simulink subsystem "EPS_Physical_Model"  (R2024a)
settings: Solver=VariableStepAuto  StartTime=0.0  StopTime=10.0  RelTol=1e-3
undefined symbols (not defined in the file): dcVoltage, Power, satellite, sensor
libraries: nesl_utility x25, fl_lib x24, ee_lib x6, autolibdatasheetbattery x1
(part 1 of 2)
settings Model: Creator=dani  LastModifiedBy=dani

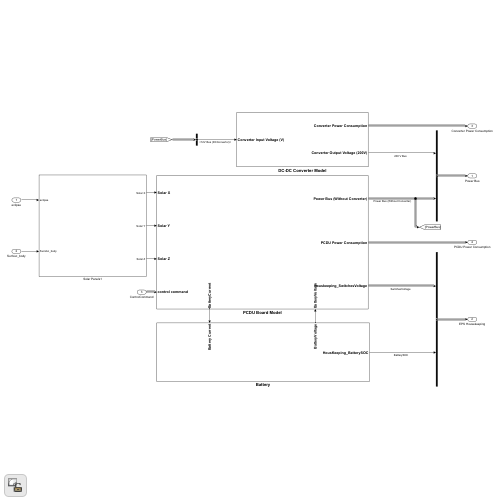
[thumbnail: Simulink's stored preview of the top-level diagram]
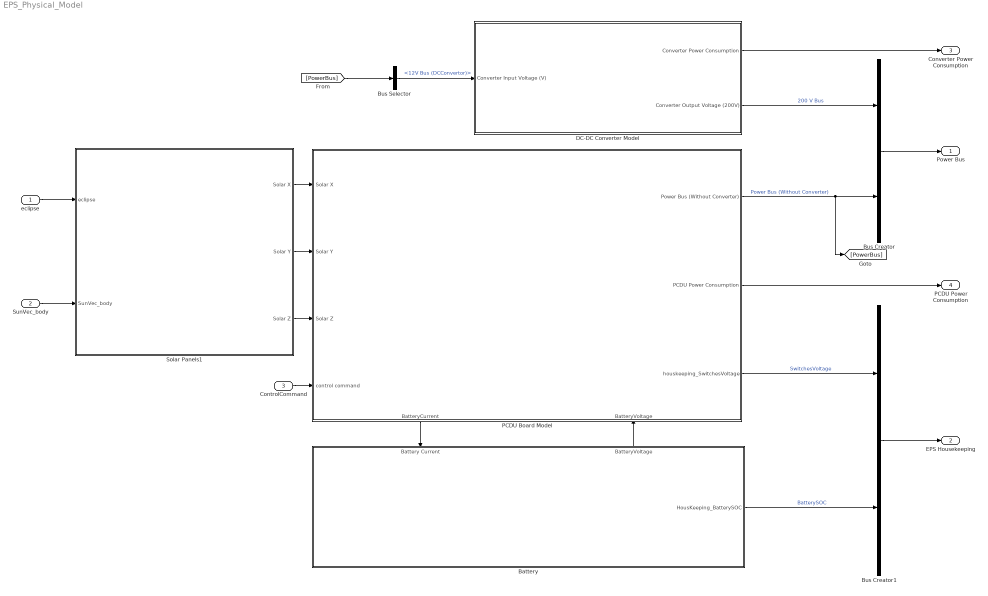
== system EPS_Physical_Model ==
  eclipse : Inport
  SunVec_body : Inport  Port=2
  ControlCommand : Inport  Port=3
  Battery : Subsystem
      settings: PortSchema="{\"entries\":[{\"content\":{\"sides\":[{\"content\":{},\"type\":\"ConnectorPlacement.EquallySpacedRectSide\",\"uuid\":\"aba023eb-c61a-4f67-b0b4-9861c526ec15\"},{\"content\":{\"connectorIds\":[\"Out1\"],\"side\":\"RIGHT\"},\"type\":\"ConnectorPlacement.EquallySpacedRectSide\",\"uuid\":\"3f6535be-9be1-4768-b763-1183b5aa3573\"},{\"content\":{\"connectorIds\":[\"In1\",\"Out2\"],\"side\":\"TOP\"},\"type\":\"ConnectorPlacement.EquallySpacedRectSide\",\"uuid\":\"4513aba4-b806-45fb-9bac-31582bd0c290\"}]},\"type\":\"ConnectorPlacement.EquallySpacedConnector\",\"uuid\":\"e35f9ef2-784c-4297-8a3a-3364ea15e971\"}],\"packageUris\":[\"http://schema.mathworks.com/mf0/Connector/R2020b\"],\"version\":\"1.0\"}"
  Bus Creator : BusCreator  Inputs=2
  Bus Creator1 : BusCreator  Inputs=2
  Bus Selector : BusSelector  OutputSignals=12V Bus (DCConvertor)
  DC-DC Converter Model : Subsystem
  PCDU Board Model : Subsystem
      settings: PortSchema="{\"entries\":[{\"content\":{\"sides\":[{\"content\":{\"connectorIds\":[\"In1\",\"In2\",\"In3\",\"In4\"]},\"type\":\"ConnectorPlacement.EquallySpacedRectSide\",\"uuid\":\"36672ca7-eb13-4725-b00c-09a487ba7d91\"},{\"content\":{\"connectorIds\":[\"Out1\",\"Out2\",\"Out3\"],\"side\":\"RIGHT\"},\"type\":\"ConnectorPlacement.EquallySpacedRectSide\",\"uuid\":\"6eafcdb3-9ad1-4020-b7cb-384bf41fe7fc\"},{\"content\":{\"side\":\"TOP\"},\"type\":\"ConnectorPlacement.EquallySpacedRectSide\",\"uuid\":\"e91cfa27-9882-4a24-903a-d0e72077027b\"},{\"content\":{\"connectorIds\":[\"Out4\",\"In5\"],\"side\":\"BOTTOM\"},\"type\":\"ConnectorPlacement.EquallySpacedRectSide\",\"uuid\":\"cff8a778-7a2c-4410-b33c-165bd9362bc6\"}]},\"type\":\"ConnectorPlacement.EquallySpacedConnector\",\"uuid\":\"92ed5259-46ff-4d91-b4a9-1e7fd77d238d\"}],\"packageUris\":[\"http://schema.mathworks.com/mf0/Connector/R2020b\"],\"version\":\"1.0\"}"
  Solar Panels1 : Subsystem
  Power Bus : Outport
  EPS Housekeeping : Outport  Port=2
  Converter Power Consumption : Outport  Port=3
  PCDU Power Consumption : Outport  Port=4
  wires:
  eclipse/1 -> Solar Panels1/1(eclipse)
  Solar Panels1/1(Solar X) -> PCDU Board Model/1(Solar X)
  Solar Panels1/2(Solar Y) -> PCDU Board Model/2(Solar Y)
  Solar Panels1/3(Solar Z) -> PCDU Board Model/3(Solar Z)
  Bus Creator/1 -> Power Bus/1
  Bus Creator1/1 -> EPS Housekeeping/1
  ControlCommand/1 -> PCDU Board Model/4(control command)
  SunVec_body/1 -> Solar Panels1/2(SunVec_body)
  PCDU Board Model/1(Power Bus (Without Converter)) -> Bus Creator/2, [PowerBus]  "Power Bus (Without Converter)"
  PCDU Board Model/4(BatteryCurrent) -> Battery/1(Battery Current)
  Battery/2(BatteryVoltage) -> PCDU Board Model/5(BatteryVoltage)
  Bus Selector/1 -> DC-DC Converter Model/1(Converter Input Voltage (V))  "<12V Bus (DCConvertor)>"
  PCDU Board Model/3(houskeeping_SwitchesVoltage) -> Bus Creator1/1  "SwitchesVoltage"
  Battery/1(HousKeeping_BatterySOC) -> Bus Creator1/2  "BatterySOC"
  [PowerBus] -> Bus Selector/1
  DC-DC Converter Model/1(Converter Power Consumption) -> Converter Power Consumption/1
  PCDU Board Model/2(PCDU Power Consumption) -> PCDU Power Consumption/1
  DC-DC Converter Model/2(Converter Output Voltage (200V)) -> Bus Creator/1  "200 V Bus"

== system EPS_Physical_Model/Battery ==
  Battery Current : Inport
  Bus Selector : BusSelector  OutputSignals=BattSoc
  Constant : Constant  Value=275
  Lithium Polymer Battery Pack : autolibdatasheetbattery/Datasheet Battery  CapacityCtrl=Parameter  OutputVlt=Unfiltered  BattChargeMax=100  Em=[2.8 3.228 3.284 3.361 3.408 3.427 3.472 3.477 3.493 3.504 3.516 3.528 3.537 3.545 3.555 3.561 3.566 3.576 3.587 3.589 3.594 3.6 3.608 3.61 3.616 3.619 3.626 3.632 3.637 3.64 3.645 3.646 3.652 3.655 3.658 3.661 3.664 3.668 3.673 3.678 3.68 3.681 3.686 3.692 3.699 3.702 3.705 3.71 3.717 3.723 3.728 3.733 3.735 3.742 3.749 3.755 3.761 3.768 3.773 3.78 3.791 3.798 3.798 3.814 3.818 3.825 3.841 3.846 3.855 3.863 3.877 3.885 3.894 3.907 3.919 3.926 3.935 3.944 3.954 3.964 3.974 3.988 3.998 4.014 4.029 4.034 4.047 4.065 4.074 4.086 4.097 4.131 4.126 4.138 4.15 4.18 4.174 4.187 4.207 4.231 4.221]  CapLUTBp=[0 0.01 0.02 0.03 0.04 0.05 0.06 0.07 0.08 0.09 0.1 0.11 0.12 0.13 0.14 0.15 0.16 0.17 0.18 0.19 0.2 0.21 0.22 0.23 0.24 0.25 0.26 0.27 0.28 0.29 0.3 0.31 0.32 0.33 0.34 0.35 0.36 0.37 0.38 0.39 0.4 0.41 0.42 0.43 0.44 0.45 0.46 0.47 0.48 0.49 0.5 0.51 0.52 0.53 0.54 0.55 0.56 0.57 0.58 0.59 0.6 0.61 0.62 0.63 0.64 0.65 0.66 0.67 0.68 0.69 0.7 0.71 0.72 0.73 0.74 0.75 0.76 0.77 0.78 0.79 0.8 0.81 0.82 0.83 0.84 0.85 0.86 0.87 0.88 0.89 0.9 0.91 0.92 0.93 0.94 0.95 0.96 0.97 0.98 0.99 1]  RInt=[0.008846 0.009319 0.009027 0.00847 0.01032 0.01314;0.006389 0.006554 0.005553 0.005525 0.006043 0.007805;0.004364 0.004101 0.00406 0.003452 0.003846 0.004517;0.002031 0.002563 0.002532 0.00246 0.002716 0.003047;0.001443 0.001825 0.001795 0.001778 0.001924 0.002234;0.0005603 0.0007192 0.0006887 0.0007557 0.0007355 0.001014;0.001028 0.001338 0.001 0.001536 0.001546 0.002789]  BattTempBp=[243.1 253.1 263.1 273.1 283.1 298.1 313.1]  CapSOCBp=[0 0.2 0.4 0.6 0.8 1]  Ns=1  Np=1  BattCapInit=100  Tc=1/1000  Vinit=4.221  RefBlkName='autolibdatasheetbattery/Datasheet Battery'
  HousKeeping_BatterySOC : Outport
  BatteryVoltage : Outport  Port=2
  wires:
  Lithium Polymer Battery Pack/2 -> BatteryVoltage/1
  Constant/1 -> Lithium Polymer Battery Pack/2
  Bus Selector/1 -> HousKeeping_BatterySOC/1  "<BattSoc>"
  Battery Current/1 -> Lithium Polymer Battery Pack/1
  Lithium Polymer Battery Pack/1 -> Bus Selector/1

== system EPS_Physical_Model/DC-DC Converter Model ==
  Converter Input Voltage (V) : Inport
  Constant : Constant  Value=satellite.Converter.OutputVoltage
  Divide : Product  Inputs=*/
  Power Consumption Calculator : Subsystem
  Product : Product
  Terminator : Terminator
  Converter Power Consumption : Outport
  Converter Output Voltage (200V) : Outport  Port=2
  wires:
  Constant/1 -> Divide/1, Converter Output Voltage (200V)/1
  Product/1 -> Terminator/1
  Power Consumption Calculator/1(Power Consumption) -> Converter Power Consumption/1
  Divide/1 -> Product/1
  Converter Input Voltage (V)/1 -> Power Consumption Calculator/1(Bus Voltage (V)), Divide/2, Product/2

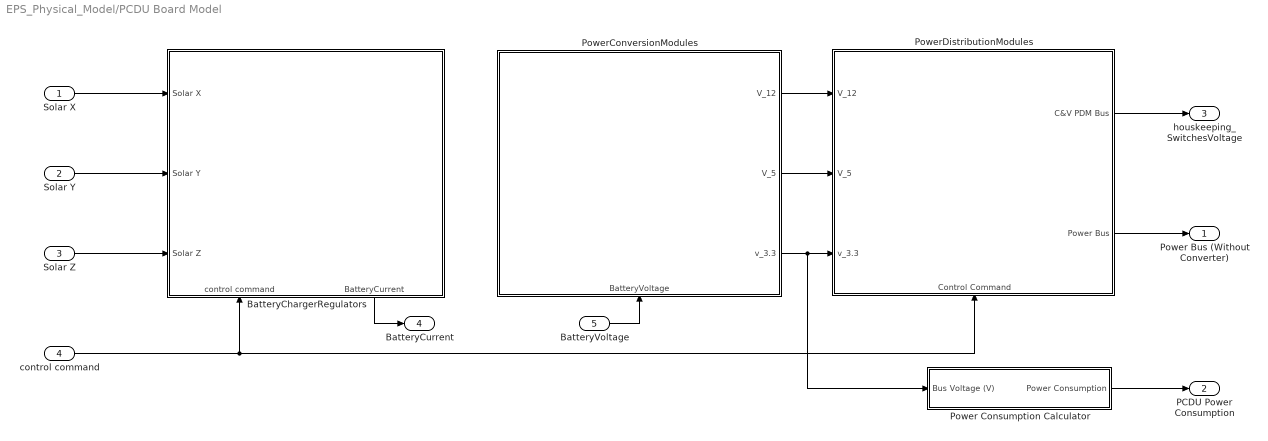
== system EPS_Physical_Model/PCDU Board Model ==
  Solar X : Inport
  Solar Y : Inport  Port=2
  Solar Z : Inport  Port=3
  control command : Inport  Port=4
  BatteryVoltage : Inport  Port=5
  BatteryChargerRegulators : Subsystem
      settings: PortSchema="{\"entries\":[{\"content\":{\"sides\":[{\"content\":{\"connectorIds\":[\"In1\",\"In2\",\"In3\"]},\"type\":\"ConnectorPlacement.EquallySpacedRectSide\",\"uuid\":\"a54c6477-f532-403d-8d22-fe8c7187031b\"},{\"content\":{\"side\":\"RIGHT\"},\"type\":\"ConnectorPlacement.EquallySpacedRectSide\",\"uuid\":\"77a78f68-d33d-41d0-b8f1-9e3ab7c3612b\"},{\"content\":{\"side\":\"TOP\"},\"type\":\"ConnectorPlacement.EquallySpacedRectSide\",\"uuid\":\"40e6fe94-fdf3-42ac-b4f7-43c530d7ca8e\"},{\"content\":{\"connectorIds\":[\"In4\",\"Out1\"],\"side\":\"BOTTOM\"},\"type\":\"ConnectorPlacement.EquallySpacedRectSide\",\"uuid\":\"5f994662-38e6-4570-aab0-67fb9122f990\"}]},\"type\":\"ConnectorPlacement.EquallySpacedConnector\",\"uuid\":\"6ae65874-5838-4158-9d12-5770a4409470\"}],\"packageUris\":[\"http://schema.mathworks.com/mf0/Connector/R2020b\"],\"version\":\"1.0\"}"
  Power Consumption Calculator : Subsystem
  PowerConversionModules : Subsystem
      settings: PortSchema="{\"entries\":[{\"content\":{\"sides\":[{\"content\":{},\"type\":\"ConnectorPlacement.EquallySpacedRectSide\",\"uuid\":\"7faa42b3-e758-4a59-bd59-cf39d4aa9549\"},{\"content\":{\"connectorIds\":[\"Out1\",\"Out2\",\"Out3\"],\"side\":\"RIGHT\"},\"type\":\"ConnectorPlacement.EquallySpacedRectSide\",\"uuid\":\"fd6f184d-0914-459d-a4a5-5106acefe1a2\"},{\"content\":{\"side\":\"TOP\"},\"type\":\"ConnectorPlacement.EquallySpacedRectSide\",\"uuid\":\"8eb7f5a0-03ff-41d6-8f99-6dc2709a1a61\"},{\"content\":{\"connectorIds\":[\"In1\"],\"side\":\"BOTTOM\"},\"type\":\"ConnectorPlacement.EquallySpacedRectSide\",\"uuid\":\"52483d8d-c391-40d7-8f9f-4b93cbeba715\"}]},\"type\":\"ConnectorPlacement.EquallySpacedConnector\",\"uuid\":\"8e205f56-f28b-497f-b412-2c567253f0db\"}],\"packageUris\":[\"http://schema.mathworks.com/mf0/Connector/R2020b\"],\"version\":\"1.0\"}"
  PowerDistributionModules : Subsystem
      settings: PortSchema="{\"entries\":[{\"content\":{\"sides\":[{\"content\":{\"connectorIds\":[\"In1\",\"In2\",\"In3\"]},\"type\":\"ConnectorPlacement.EquallySpacedRectSide\",\"uuid\":\"cc944067-0ae4-44c1-82d9-a1ec81fe8cae\"},{\"content\":{\"connectorIds\":[\"Out1\",\"Out2\"],\"side\":\"RIGHT\"},\"type\":\"ConnectorPlacement.EquallySpacedRectSide\",\"uuid\":\"14a8b3bc-9f23-4806-a571-fc273ce75e66\"},{\"content\":{\"side\":\"TOP\"},\"type\":\"ConnectorPlacement.EquallySpacedRectSide\",\"uuid\":\"d74dfaa3-3ba0-49fd-a7b0-c7f12b34c19f\"},{\"content\":{\"connectorIds\":[\"In4\"],\"side\":\"BOTTOM\"},\"type\":\"ConnectorPlacement.EquallySpacedRectSide\",\"uuid\":\"4657f579-020f-4b4b-b590-abcb58cae511\"}]},\"type\":\"ConnectorPlacement.EquallySpacedConnector\",\"uuid\":\"36922770-3f3d-4d84-84df-ae2b6fb05eab\"}],\"packageUris\":[\"http://schema.mathworks.com/mf0/Connector/R2020b\"],\"version\":\"1.0\"}"
  Power Bus (Without Converter) : Outport
  PCDU Power Consumption : Outport  Port=2
  houskeeping_SwitchesVoltage : Outport  Port=3
  BatteryCurrent : Outport  Port=4
  wires:
  control command/1 -> BatteryChargerRegulators/4(control command), PowerDistributionModules/4(Control Command)
  PowerConversionModules/2(V_5) -> PowerDistributionModules/2(V_5)
  PowerConversionModules/1(V_12) -> PowerDistributionModules/1(V_12)
  BatteryVoltage/1 -> PowerConversionModules/1(BatteryVoltage)
  PowerConversionModules/3(v_3.3) -> PowerDistributionModules/3(v_3.3), Power Consumption Calculator/1(Bus Voltage (V))
  BatteryChargerRegulators/1(BatteryCurrent) -> BatteryCurrent/1
  Power Consumption Calculator/1(Power Consumption) -> PCDU Power Consumption/1
  PowerDistributionModules/1(C&V PDM Bus) -> houskeeping_SwitchesVoltage/1
  Solar Y/1 -> BatteryChargerRegulators/2(Solar Y)
  PowerDistributionModules/2(Power Bus) -> Power Bus (Without Converter)/1
  Solar Z/1 -> BatteryChargerRegulators/3(Solar Z)
  Solar X/1 -> BatteryChargerRegulators/1(Solar X)

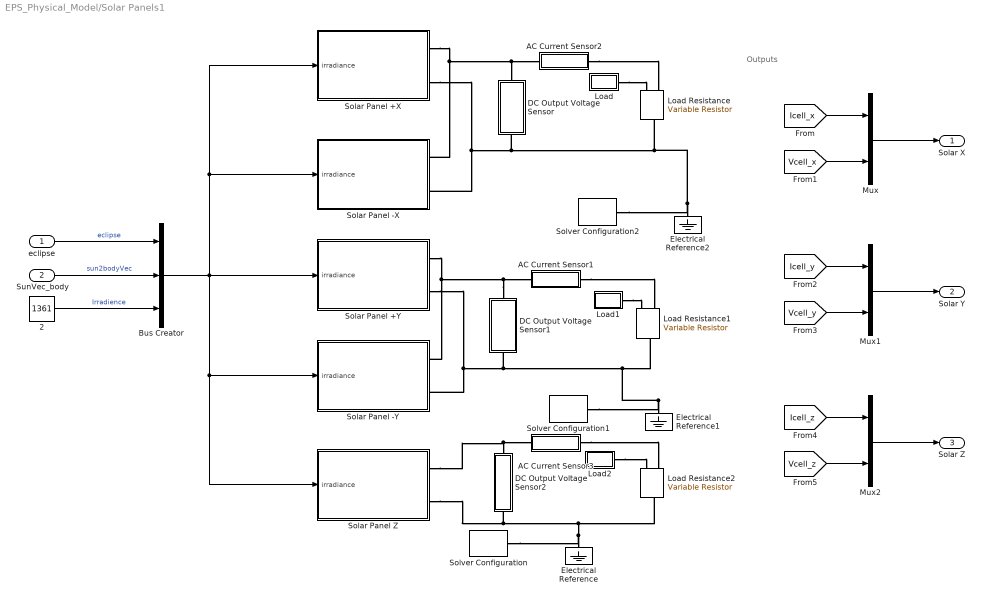
== system EPS_Physical_Model/Solar Panels1 ==
  note: Outputs
  eclipse : Inport
  SunVec_body : Inport  Port=2
  " 2" : Constant  Value=1361
  AC Current Sensor1 : Subsystem
      mask Display: disp('i');
  AC Current Sensor2 : Subsystem
      mask Display: disp('i');
  AC Current Sensor3 : Subsystem
      mask Display: disp('i');
  Bus Creator : BusCreator  Inputs=3
  DC Output Voltage Sensor : Subsystem
      mask Display: disp('v')
  DC Output Voltage Sensor1 : Subsystem
      mask Display: disp('v')
  DC Output Voltage Sensor2 : Subsystem
      mask Display: disp('v')
  Electrical Reference : fl_lib/Electrical/Electrical Elements/Electrical Reference
  Electrical Reference1 : fl_lib/Electrical/Electrical Elements/Electrical Reference
  Electrical Reference2 : fl_lib/Electrical/Electrical Elements/Electrical Reference
  Load : Subsystem
  Load Resistance : fl_lib/Electrical/Electrical Elements/Variable Resistor  Rmin=0 Ohm  thermalEnable=false  thermal_mass=1 J/K  i_specify=off  i_priority=None  i=5 A  i_nominal_specify=off  i_nominal_value=1  i_nominal_unit=A  v_specify=off  v_priority=None  v=0 V  v_nominal_specify=off  v_nominal_value=1  v_nominal_unit=V  T_specify=off  T_priority=None  T=300 K  T_nominal_specify=off  T_nominal_value=1  T_nominal_unit=K
  Load Resistance1 : fl_lib/Electrical/Electrical Elements/Variable Resistor  Rmin=0 Ohm  thermalEnable=false  thermal_mass=1 J/K  i_specify=off  i_priority=None  i=5 A  i_nominal_specify=off  i_nominal_value=1  i_nominal_unit=A  v_specify=off  v_priority=None  v=0 V  v_nominal_specify=off  v_nominal_value=1  v_nominal_unit=V  T_specify=off  T_priority=None  T=300 K  T_nominal_specify=off  T_nominal_value=1  T_nominal_unit=K
  Load Resistance2 : fl_lib/Electrical/Electrical Elements/Variable Resistor  Rmin=0 Ohm  thermalEnable=false  thermal_mass=1 J/K  i_specify=off  i_priority=None  i=5 A  i_nominal_specify=off  i_nominal_value=1  i_nominal_unit=A  v_specify=off  v_priority=None  v=0 V  v_nominal_specify=off  v_nominal_value=1  v_nominal_unit=V  T_specify=off  T_priority=None  T=300 K  T_nominal_specify=off  T_nominal_value=1  T_nominal_unit=K
  Load1 : Subsystem
  Load2 : Subsystem
  Mux : Mux  Inputs=2
  Mux1 : Mux  Inputs=2
  Mux2 : Mux  Inputs=2
  Solar Panel +X : Subsystem
  Solar Panel +Y : Subsystem
  Solar Panel -X : Subsystem
  Solar Panel -Y : Subsystem
  Solar Panel Z : Subsystem
  Solver Configuration : nesl_utility/Solver Configuration  PhysicalDomain=network_engine_domain  SubClassName=solver  LeftPortType=input  RightPortType=generic  Tones=[]  Harmonics=[]  SimulateNoise=off  Profile=off  UseLocalSampling=off  EnableSwitchedLinearOptims=on  FrequencyDomain=off  UseCCode=off  RelTol=0.001  AbsTol=0.001  MinStep=1e-09  ToWorkspace=off  RevertToSquareIcSolve=off  NumHomotopyIterations=100  PhasorMode=off  PhasorModeNumHarmonics=1  ConsistencySolver=NEWTON_XTOL_AFTER_FTOL  IndexReductionMethod=DerivativeReplacement  DoDC=off  ResidualTolerance=1e-09  ConsistencyTolSource=GLOBAL  ConsistencyAbsTol=0.001  ConsistencyRelTol=0.001  ConsistencyTolFactor=0.001  UseLocalSolver=off  LocalSolverChoice=NE_BACKWARD_EULER_ADVANCER  ResolveIndetEquations=on  FunctionEvalNumThread=1  LocalSolverSampleTime=0.001  DoFixedCost=off  MaxNonlinIter=3  MaxModeIter=2  ComputeImpulses=off  ImpulseIterations=2  LinearAlgebra=auto  LinearAlgebraNumThread=0  EquationFormulation=NE_TIME_EF  DelaysMemoryBudget=1024  AutomaticFiltering=on  FilteringTimeConstant=0.001  PartitionStorageMethod=AS_NEEDED  PartitionMemoryBudget=1024  PartitionMethod=ROBUST  MultibodyUseLocalSolver=off  MultibodyLocalSolverChoice=ODE1  MultibodyLocalSolverSampleTime=0.001
  Solver Configuration1 : nesl_utility/Solver Configuration  PhysicalDomain=network_engine_domain  SubClassName=solver  LeftPortType=input  RightPortType=generic  Tones=[]  Harmonics=[]  SimulateNoise=off  Profile=off  UseLocalSampling=off  EnableSwitchedLinearOptims=on  FrequencyDomain=off  UseCCode=off  RelTol=0.001  AbsTol=0.001  MinStep=1e-09  ToWorkspace=off  RevertToSquareIcSolve=off  NumHomotopyIterations=100  PhasorMode=off  PhasorModeNumHarmonics=1  ConsistencySolver=NEWTON_XTOL_AFTER_FTOL  IndexReductionMethod=DerivativeReplacement  DoDC=off  ResidualTolerance=1e-09  ConsistencyTolSource=GLOBAL  ConsistencyAbsTol=0.001  ConsistencyRelTol=0.001  ConsistencyTolFactor=0.001  UseLocalSolver=off  LocalSolverChoice=NE_BACKWARD_EULER_ADVANCER  ResolveIndetEquations=on  FunctionEvalNumThread=1  LocalSolverSampleTime=0.001  DoFixedCost=off  MaxNonlinIter=3  MaxModeIter=2  ComputeImpulses=off  ImpulseIterations=2  LinearAlgebra=auto  LinearAlgebraNumThread=0  EquationFormulation=NE_TIME_EF  DelaysMemoryBudget=1024  AutomaticFiltering=on  FilteringTimeConstant=0.001  PartitionStorageMethod=AS_NEEDED  PartitionMemoryBudget=1024  PartitionMethod=ROBUST  MultibodyUseLocalSolver=off  MultibodyLocalSolverChoice=ODE1  MultibodyLocalSolverSampleTime=0.001
  Solver Configuration2 : nesl_utility/Solver Configuration  PhysicalDomain=network_engine_domain  SubClassName=solver  LeftPortType=input  RightPortType=generic  Tones=[]  Harmonics=[]  SimulateNoise=off  Profile=off  UseLocalSampling=off  EnableSwitchedLinearOptims=on  FrequencyDomain=off  UseCCode=off  RelTol=0.001  AbsTol=0.001  MinStep=1e-09  ToWorkspace=off  RevertToSquareIcSolve=off  NumHomotopyIterations=100  PhasorMode=off  PhasorModeNumHarmonics=1  ConsistencySolver=NEWTON_XTOL_AFTER_FTOL  IndexReductionMethod=DerivativeReplacement  DoDC=off  ResidualTolerance=1e-09  ConsistencyTolSource=GLOBAL  ConsistencyAbsTol=0.001  ConsistencyRelTol=0.001  ConsistencyTolFactor=0.001  UseLocalSolver=off  LocalSolverChoice=NE_BACKWARD_EULER_ADVANCER  ResolveIndetEquations=on  FunctionEvalNumThread=1  LocalSolverSampleTime=0.001  DoFixedCost=off  MaxNonlinIter=3  MaxModeIter=2  ComputeImpulses=off  ImpulseIterations=2  LinearAlgebra=auto  LinearAlgebraNumThread=0  EquationFormulation=NE_TIME_EF  DelaysMemoryBudget=1024  AutomaticFiltering=on  FilteringTimeConstant=0.001  PartitionStorageMethod=AS_NEEDED  PartitionMemoryBudget=1024  PartitionMethod=ROBUST  MultibodyUseLocalSolver=off  MultibodyLocalSolverChoice=ODE1  MultibodyLocalSolverSampleTime=0.001
  Solar X : Outport
  Solar Y : Outport  Port=2
  Solar Z : Outport  Port=3
  wires:
  SunVec_body/1 -> Bus Creator/2  "sun2bodyVec"
  eclipse/1 -> Bus Creator/1  "eclipse"
  " 2"/1 -> Bus Creator/3  "Irradience"
  Mux1/1 -> Solar Y/1
  Mux2/1 -> Solar Z/1
  Mux/1 -> Solar X/1
  [Vcell_z] -> Mux2/2
  [Icell_z] -> Mux2/1
  [Icell_x] -> Mux/1
  [Vcell_x] -> Mux/2
  [Icell_y] -> Mux1/1
  [Vcell_y] -> Mux1/2
  Bus Creator/1 -> Solar Panel +Y/1(irradiance), Solar Panel Z/1(irradiance), Solar Panel -Y/1(irradiance), Solar Panel +X/1(irradiance), Solar Panel -X/1(irradiance)
  connections:
  AC Current Sensor2/LConn1 -- Load Resistance/LConn2
  Load1/RConn1 -- Load Resistance1/LConn1
  Load2/RConn1 -- Load Resistance2/LConn1
  AC Current Sensor1/LConn1 -- Load Resistance1/LConn2
  Load/RConn1 -- Load Resistance/LConn1
  AC Current Sensor3/LConn1 -- Load Resistance2/LConn2
  DC Output Voltage Sensor2/RConn1 -- Solar Panel Z/RConn1 -- AC Current Sensor3/RConn1
  Solver Configuration1/RConn1 -- DC Output Voltage Sensor1/LConn1 -- Solar Panel -Y/RConn2 -- Solar Panel +Y/RConn2 -- Load Resistance1/RConn1 -- Electrical Reference1/LConn1
  Load Resistance2/RConn1 -- Electrical Reference/LConn1 -- Solver Configuration/RConn1 -- Solar Panel Z/RConn2 -- DC Output Voltage Sensor2/LConn1
  Solar Panel -X/RConn1 -- Solar Panel +X/RConn1 -- AC Current Sensor2/RConn1 -- DC Output Voltage Sensor/RConn1
  Solver Configuration2/RConn1 -- Load Resistance/RConn1 -- Solar Panel -X/RConn2 -- Solar Panel +X/RConn2 -- DC Output Voltage Sensor/LConn1 -- Electrical Reference2/LConn1
  DC Output Voltage Sensor1/RConn1 -- AC Current Sensor1/RConn1 -- Solar Panel -Y/RConn1 -- Solar Panel +Y/RConn1

== system EPS_Physical_Model/DC-DC Converter Model/Power Consumption Calculator ==
  note: $I_=\frac{V_{Bus}}{R} \\ P_{Consumption} =I V_{Bus}$
  Bus Voltage (V) : Inport
  1/R : Gain  Gain=1/Power.Converter.Resistance
  Bus Creator : BusCreator  Inputs=2
  Product : Product
  Power Consumption : Outport
  wires:
  Product/1 -> Bus Creator/2  "Power Consumption (W)"
  Bus Creator/1 -> Power Consumption/1
  1/R/1 -> Bus Creator/1, Product/1  "Current (A)"
  Bus Voltage (V)/1 -> 1/R/1, Product/2

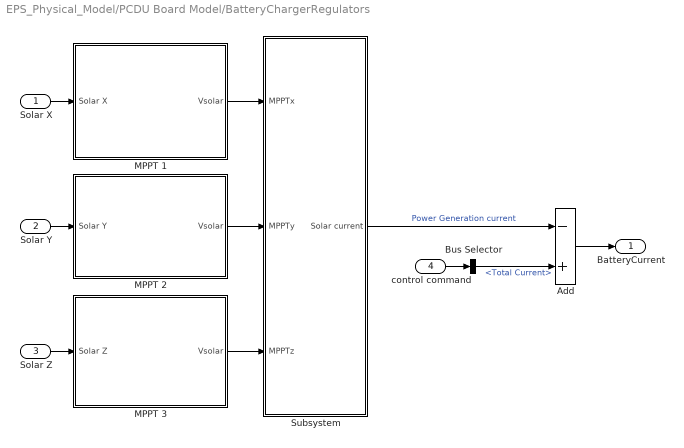
== system EPS_Physical_Model/PCDU Board Model/BatteryChargerRegulators ==
  Solar X : Inport
  Solar Y : Inport  Port=2
  Solar Z : Inport  Port=3
  control command : Inport  Port=4
  Add : Sum  Inputs=-+
  Bus Selector : BusSelector  OutputSignals=Total Current
  MPPT 1 : Subsystem
  MPPT 2 : Subsystem
  MPPT 3 : Subsystem
  Subsystem : Subsystem
  BatteryCurrent : Outport
  wires:
  control command/1 -> Bus Selector/1
  Bus Selector/1 -> Add/2  "<Total Current>"
  Solar Z/1 -> MPPT 3/1(Solar Z)
  Solar X/1 -> MPPT 1/1(Solar X)
  MPPT 3/1(Vsolar) -> Subsystem/3(MPPTz)
  Subsystem/1(Solar current) -> Add/1  "Power Generation current"
  Solar Y/1 -> MPPT 2/1(Solar Y)
  MPPT 1/1(Vsolar) -> Subsystem/1(MPPTx)
  Add/1 -> BatteryCurrent/1
  MPPT 2/1(Vsolar) -> Subsystem/2(MPPTy)

== system EPS_Physical_Model/PCDU Board Model/Power Consumption Calculator ==
  note: $I_=\frac{V_{Bus}}{R} \\ P_{Consumption} =I V_{Bus}$
  Bus Voltage (V) : Inport
  1/R : Gain  Gain=1/Power.PCDU.Resistance
  Bus Creator : BusCreator  Inputs=2
  Product : Product
  Power Consumption : Outport
  wires:
  Product/1 -> Bus Creator/2  "Power Consumption (W)"
  Bus Creator/1 -> Power Consumption/1
  1/R/1 -> Bus Creator/1, Product/1  "Current (A)"
  Bus Voltage (V)/1 -> 1/R/1, Product/2

== system EPS_Physical_Model/PCDU Board Model/PowerConversionModules ==
  BatteryVoltage : Inport
  Boost_12V : Subsystem
  Boost_3.3V : Subsystem
  Boost_5V : Subsystem
  V_12 : Outport
  V_5 : Outport  Port=2
  v_3.3 : Outport  Port=3
  wires:
  Boost_3.3V/1(12V) -> v_3.3/1
  Boost_5V/1(12V) -> V_5/1
  Boost_12V/1(12V) -> V_12/1
  BatteryVoltage/1 -> Boost_5V/1(BatteryVoltage), Boost_3.3V/1(BatteryVoltage), Boost_12V/1(BatteryVoltage)

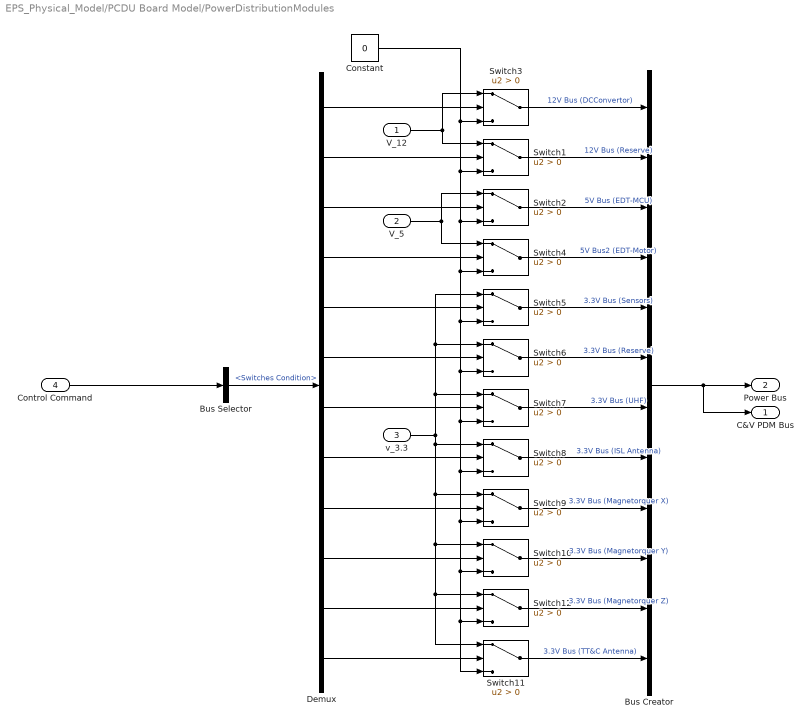
== system EPS_Physical_Model/PCDU Board Model/PowerDistributionModules ==
  V_12 : Inport
  V_5 : Inport  Port=2
  v_3.3 : Inport  Port=3
  Control Command : Inport  Port=4
  Bus Creator : BusCreator  Inputs=12
  Bus Selector : BusSelector  OutputSignals=Switches Condition
  Constant : Constant  Value=0
  Demux : Demux  Outputs=12
  Switch{1..12} (12 alike) : Switch  Criteria=u2 > Threshold  SaturateOnIntegerOverflow=off  InputSameDT=off
  C&V PDM Bus : Outport
  Power Bus : Outport  Port=2
  wires:
  Bus Selector/1 -> Demux/1  "<Switches Condition>"
  Demux/12 -> Switch11/2
  Demux/11 -> Switch12/2
  Demux/10 -> Switch10/2
  Demux/9 -> Switch9/2
  Demux/8 -> Switch8/2
  Demux/7 -> Switch7/2
  Demux/6 -> Switch6/2
  Demux/5 -> Switch5/2
  Demux/4 -> Switch4/2
  Demux/3 -> Switch2/2
  Demux/2 -> Switch1/2
  Demux/1 -> Switch3/2
  Bus Creator/1 -> C&V PDM Bus/1, Power Bus/1
  Switch11/1 -> Bus Creator/12  "3.3V Bus (TT&C Antenna)"
  Switch12/1 -> Bus Creator/11  "3.3V Bus (Magnetorquer Z)"
  Switch10/1 -> Bus Creator/10  "3.3V Bus (Magnetorquer Y)"
  Switch9/1 -> Bus Creator/9  "3.3V Bus (Magnetorquer X)"
  Switch8/1 -> Bus Creator/8  "3.3V Bus (ISL Antenna)"
  Switch7/1 -> Bus Creator/7  "3.3V Bus (UHF)"
  Switch6/1 -> Bus Creator/6  "3.3V Bus (Reserve)"
  Switch5/1 -> Bus Creator/5  "3.3V Bus (Sensors)"
  Switch4/1 -> Bus Creator/4  "5V Bus2 (EDT-Motor)"
  Switch2/1 -> Bus Creator/3  "5V Bus (EDT-MCU)"
  Switch1/1 -> Bus Creator/2  "12V Bus (Reserve)"
  Switch3/1 -> Bus Creator/1  "12V Bus (DCConvertor)"
  v_3.3/1 -> Switch8/1, Switch9/1, Switch10/1, Switch12/1, Switch11/1, Switch5/1, Switch6/1, Switch7/1
  V_5/1 -> Switch2/1, Switch4/1
  V_12/1 -> Switch3/1, Switch1/1
  Control Command/1 -> Bus Selector/1
  Constant/1 -> Switch3/3, Switch1/3, Switch2/3, Switch4/3, Switch5/3, Switch6/3, Switch7/3, Switch8/3, Switch9/3, Switch10/3, Switch12/3, Switch11/3

== system EPS_Physical_Model/Solar Panels1/AC Current Sensor1 ==
  Current Sensor : fl_lib/Electrical/Electrical Sensors/Current Sensor
  PS-Simulink Converter : nesl_utility/PS-Simulink Converter  PhysicalDomain=network_engine_domain  SubClassName=ps_output  LeftPortType=input  RightPortType=output  PseudoPeriodic=off  Frequencies=[]  VectorFormat=1-D array  Unit=1  AffineConversion=off
  Sensor dynamics : TransferFcn  Numerator=1  Denominator=[1 1]
  - : PMIOPort  Side=Left
  + : PMIOPort  Port=2  Side=Right
  tag scope: Icell_y=global
  wires:
  PS-Simulink Converter/1 -> Sensor dynamics/1
  Sensor dynamics/1 -> [Icell_y]
  connections:
  Current Sensor/RConn1 -- PS-Simulink Converter/LConn1
  +/RConn1 -- Current Sensor/LConn1
  Current Sensor/RConn2 -- -/RConn1

== system EPS_Physical_Model/Solar Panels1/AC Current Sensor2 ==
  Current Sensor : fl_lib/Electrical/Electrical Sensors/Current Sensor
  PS-Simulink Converter : nesl_utility/PS-Simulink Converter  PhysicalDomain=network_engine_domain  SubClassName=ps_output  LeftPortType=input  RightPortType=output  PseudoPeriodic=off  Frequencies=[]  VectorFormat=1-D array  Unit=1  AffineConversion=off
  Sensor dynamics : TransferFcn  Numerator=1  Denominator=[1 1]
  - : PMIOPort  Side=Left
  + : PMIOPort  Port=2  Side=Right
  tag scope: Icell_x=global
  wires:
  Sensor dynamics/1 -> [Icell_x]
  PS-Simulink Converter/1 -> Sensor dynamics/1
  connections:
  Current Sensor/RConn2 -- -/RConn1
  +/RConn1 -- Current Sensor/LConn1
  Current Sensor/RConn1 -- PS-Simulink Converter/LConn1

== system EPS_Physical_Model/Solar Panels1/AC Current Sensor3 ==
  Current Sensor : fl_lib/Electrical/Electrical Sensors/Current Sensor
  PS-Simulink Converter : nesl_utility/PS-Simulink Converter  PhysicalDomain=network_engine_domain  SubClassName=ps_output  LeftPortType=input  RightPortType=output  PseudoPeriodic=off  Frequencies=[]  VectorFormat=1-D array  Unit=1  AffineConversion=off
  Sensor dynamics : TransferFcn  Numerator=1  Denominator=[1 1]
  Solver Configuration : nesl_utility/Solver Configuration  Commented=on  PhysicalDomain=network_engine_domain  SubClassName=solver  LeftPortType=input  RightPortType=generic  Tones=[]  Harmonics=[]  SimulateNoise=off  Profile=off  UseLocalSampling=off  EnableSwitchedLinearOptims=on  FrequencyDomain=off  UseCCode=off  RelTol=0.001  AbsTol=0.001  MinStep=1e-09  ToWorkspace=off  RevertToSquareIcSolve=off  NumHomotopyIterations=100  PhasorMode=off  PhasorModeNumHarmonics=1  ConsistencySolver=NEWTON_XTOL_AFTER_FTOL  IndexReductionMethod=DerivativeReplacement  DoDC=off  ResidualTolerance=1e-09  ConsistencyTolSource=GLOBAL  ConsistencyAbsTol=0.001  ConsistencyRelTol=0.001  ConsistencyTolFactor=0.001  UseLocalSolver=off  LocalSolverChoice=NE_PARTITIONING_ADVANCER  ResolveIndetEquations=on  FunctionEvalNumThread=1  LocalSolverSampleTime=0.001  DoFixedCost=on  MaxNonlinIter=3  MaxModeIter=2  ComputeImpulses=off  ImpulseIterations=2  LinearAlgebra=auto  LinearAlgebraNumThread=0  EquationFormulation=NE_TIME_EF  DelaysMemoryBudget=1024  AutomaticFiltering=on  FilteringTimeConstant=0.001  PartitionStorageMethod=AS_NEEDED  PartitionMemoryBudget=1024  PartitionMethod=FAST  MultibodyUseLocalSolver=off  MultibodyLocalSolverChoice=ODE1  MultibodyLocalSolverSampleTime=0.001
  - : PMIOPort  Side=Left
  + : PMIOPort  Port=2  Side=Right
  tag scope: Icell_z=global
  wires:
  Sensor dynamics/1 -> [Icell_z]
  PS-Simulink Converter/1 -> Sensor dynamics/1
  connections:
  Current Sensor/RConn2 -- -/RConn1
  Current Sensor/LConn1 -- Solver Configuration/RConn1 -- +/RConn1
  Current Sensor/RConn1 -- PS-Simulink Converter/LConn1

== system EPS_Physical_Model/Solar Panels1/DC Output Voltage Sensor ==
  PS-Simulink Converter : nesl_utility/PS-Simulink Converter  PhysicalDomain=network_engine_domain  SubClassName=ps_output  LeftPortType=input  RightPortType=output  PseudoPeriodic=off  Frequencies=[]  VectorFormat=1-D array  Unit=1  AffineConversion=off
  Sensor dynamics : TransferFcn  Numerator=1  Denominator=[1 1]
  Voltage Sensor : fl_lib/Electrical/Electrical Sensors/Voltage Sensor
  - : PMIOPort  Side=Left
  + : PMIOPort  Port=2  Side=Right
  tag scope: Vcell_x=global
  wires:
  Sensor dynamics/1 -> [Vcell_x]
  PS-Simulink Converter/1 -> Sensor dynamics/1
  connections:
  Voltage Sensor/LConn1 -- +/RConn1
  Voltage Sensor/RConn1 -- PS-Simulink Converter/LConn1
  Voltage Sensor/RConn2 -- -/RConn1

== system EPS_Physical_Model/Solar Panels1/DC Output Voltage Sensor1 ==
  PS-Simulink Converter : nesl_utility/PS-Simulink Converter  PhysicalDomain=network_engine_domain  SubClassName=ps_output  LeftPortType=input  RightPortType=output  PseudoPeriodic=off  Frequencies=[]  VectorFormat=1-D array  Unit=1  AffineConversion=off
  Sensor dynamics : TransferFcn  Numerator=1  Denominator=[1 1]
  Voltage Sensor : fl_lib/Electrical/Electrical Sensors/Voltage Sensor
  - : PMIOPort  Side=Left
  + : PMIOPort  Port=2  Side=Right
  tag scope: Vcell_y=global
  wires:
  PS-Simulink Converter/1 -> Sensor dynamics/1
  Sensor dynamics/1 -> [Vcell_y]
  connections:
  Voltage Sensor/RConn2 -- -/RConn1
  Voltage Sensor/RConn1 -- PS-Simulink Converter/LConn1
  Voltage Sensor/LConn1 -- +/RConn1

== system EPS_Physical_Model/Solar Panels1/DC Output Voltage Sensor2 ==
  PS-Simulink Converter : nesl_utility/PS-Simulink Converter  PhysicalDomain=network_engine_domain  SubClassName=ps_output  LeftPortType=input  RightPortType=output  PseudoPeriodic=off  Frequencies=[]  VectorFormat=1-D array  Unit=1  AffineConversion=off
  Sensor dynamics : TransferFcn  Numerator=1  Denominator=[1 1]
  Voltage Sensor : fl_lib/Electrical/Electrical Sensors/Voltage Sensor
  - : PMIOPort  Side=Left
  + : PMIOPort  Port=2  Side=Right
  tag scope: Vcell_z=global
  wires:
  Sensor dynamics/1 -> [Vcell_z]
  PS-Simulink Converter/1 -> Sensor dynamics/1
  connections:
  Voltage Sensor/LConn1 -- +/RConn1
  Voltage Sensor/RConn1 -- PS-Simulink Converter/LConn1
  Voltage Sensor/RConn2 -- -/RConn1

== system EPS_Physical_Model/Solar Panels1/Load ==
  " " : Constant
  " 1" : Constant  Value=1.5
  Constant : Constant  Value=5
  Load Power (kW) : Gain  Gain=1.688857025146485
  Simulink-PS Converter1 : nesl_utility/Simulink-PS Converter  PhysicalDomain=network_engine_domain  SubClassName=ps_input  LeftPortType=input  RightPortType=output  PseudoPeriodic=off  Frequencies=[]  NoiseDistribution=none  NoiseParameters=[]  Unit=1  AffineConversion=off  FilteringAndDerivatives=provide  SimscapeFilterOrder=1  InputFilterTimeConstant=0.001  UdotUserProvided=0
  Switch : Switch  Criteria=u2 > Threshold  SaturateOnIntegerOverflow=off  InputSameDT=off
  V^2/P : Product  Inputs=*/
  kW2W : Gain  Gain=1000
  R : PMIOPort  Side=Right
  wires:
  kW2W/1 -> V^2/P/2
  Switch/1 -> kW2W/1
  V^2/P/1 -> Simulink-PS Converter1/1
  Constant/1 -> V^2/P/1
  " 1"/1 -> Switch/3
  Load Power (kW)/1 -> Switch/2, Switch/1
  " "/1 -> Load Power (kW)/1
  connections:
  Simulink-PS Converter1/RConn1 -- R/RConn1

== system EPS_Physical_Model/Solar Panels1/Load1 ==
  " " : Constant
  " 1" : Constant  Value=1.5
  Constant : Constant  Value=5
  Load Power (kW) : Gain  Gain=1.688857025146485
  Simulink-PS Converter1 : nesl_utility/Simulink-PS Converter  PhysicalDomain=network_engine_domain  SubClassName=ps_input  LeftPortType=input  RightPortType=output  PseudoPeriodic=off  Frequencies=[]  NoiseDistribution=none  NoiseParameters=[]  Unit=1  AffineConversion=off  FilteringAndDerivatives=provide  SimscapeFilterOrder=1  InputFilterTimeConstant=0.001  UdotUserProvided=0
  Switch : Switch  Criteria=u2 > Threshold  SaturateOnIntegerOverflow=off  InputSameDT=off
  V^2/P : Product  Inputs=*/
  kW2W : Gain  Gain=1000
  R : PMIOPort  Side=Right
  wires:
  " "/1 -> Load Power (kW)/1
  Load Power (kW)/1 -> Switch/1, Switch/2
  " 1"/1 -> Switch/3
  Constant/1 -> V^2/P/1
  V^2/P/1 -> Simulink-PS Converter1/1
  Switch/1 -> kW2W/1
  kW2W/1 -> V^2/P/2
  connections:
  Simulink-PS Converter1/RConn1 -- R/RConn1

== system EPS_Physical_Model/Solar Panels1/Load2 ==
  " " : Constant
  " 1" : Constant  Value=1.5
  Constant : Constant  Value=5
  Load Power (kW) : Gain  Gain=1.688857025146485
  Simulink-PS Converter1 : nesl_utility/Simulink-PS Converter  PhysicalDomain=network_engine_domain  SubClassName=ps_input  LeftPortType=input  RightPortType=output  PseudoPeriodic=off  Frequencies=[]  NoiseDistribution=none  NoiseParameters=[]  Unit=1  AffineConversion=off  FilteringAndDerivatives=provide  SimscapeFilterOrder=1  InputFilterTimeConstant=0.001  UdotUserProvided=0
  Switch : Switch  Criteria=u2 > Threshold  SaturateOnIntegerOverflow=off  InputSameDT=off
  V^2/P : Product  Inputs=*/
  kW2W : Gain  Gain=1000
  R : PMIOPort  Side=Right
  wires:
  kW2W/1 -> V^2/P/2
  Switch/1 -> kW2W/1
  V^2/P/1 -> Simulink-PS Converter1/1
  Constant/1 -> V^2/P/1
  " 1"/1 -> Switch/3
  Load Power (kW)/1 -> Switch/2, Switch/1
  " "/1 -> Load Power (kW)/1
  connections:
  Simulink-PS Converter1/RConn1 -- R/RConn1

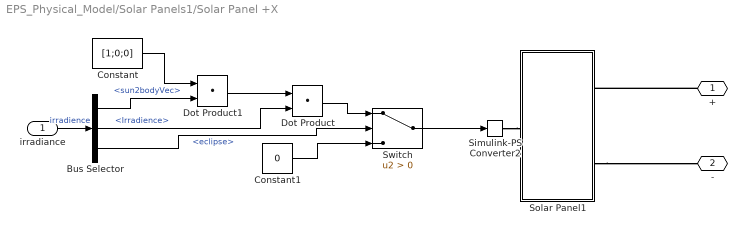
== system EPS_Physical_Model/Solar Panels1/Solar Panel +X ==
  irradiance : Inport
  Bus Selector : BusSelector  OutputSignals=sun2bodyVec,Irradience,eclipse
  Constant : Constant  Value=[1;0;0]
  Constant1 : Constant  Value=0
  Dot Product : DotProduct  OutDataTypeStr=Inherit: Inherit via internal rule
  Dot Product1 : DotProduct  OutDataTypeStr=Inherit: Inherit via internal rule
  Simulink-PS Converter2 : nesl_utility/Simulink-PS Converter  PhysicalDomain=network_engine_domain  SubClassName=ps_input  LeftPortType=input  RightPortType=output  PseudoPeriodic=off  Frequencies=[]  NoiseDistribution=none  NoiseParameters=[]  Unit=1  AffineConversion=off  FilteringAndDerivatives=filter  SimscapeFilterOrder=1  InputFilterTimeConstant=0.001  UdotUserProvided=0
  Solar Panel1 : Subsystem  mask(Solar Panel){}
      mask help: Models a solar panel using a parallel-connected string of solar cells. The solar cell strings are modeled using a single Solar Cell block from the Simscape(TM) Electrical(TM) Sources library.
      mask Display: image('ee_solar_panel_icon.jpg')
  Switch : Switch  Criteria=u2 > Threshold  SaturateOnIntegerOverflow=off  InputSameDT=off
  + : PMIOPort  Side=Right
  - : PMIOPort  Port=2  Side=Right
  wires:
  Bus Selector/1 -> Dot Product1/2  "<sun2bodyVec>"
  Bus Selector/2 -> Dot Product/2  "<Irradience>"
  Bus Selector/3 -> Switch/2  "<eclipse>"
  Constant1/1 -> Switch/3
  Dot Product/1 -> Switch/1
  Switch/1 -> Simulink-PS Converter2/1
  Constant/1 -> Dot Product1/1
  Dot Product1/1 -> Dot Product/1
  irradiance/1 -> Bus Selector/1  "irradience"
  connections:
  Solar Panel1/RConn2 -- -/RConn1
  +/RConn1 -- Solar Panel1/RConn1
  Simulink-PS Converter2/RConn1 -- Solar Panel1/LConn1

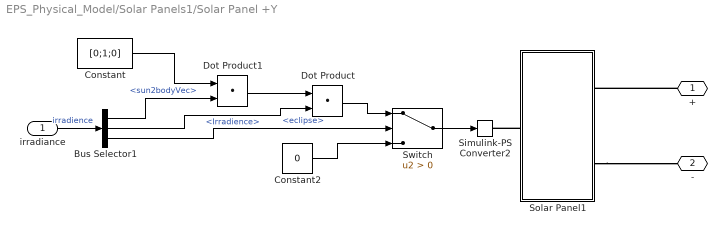
== system EPS_Physical_Model/Solar Panels1/Solar Panel +Y ==
  irradiance : Inport
  Bus Selector1 : BusSelector  OutputSignals=sun2bodyVec,Irradience,eclipse
  Constant : Constant  Value=[0;1;0]
  Constant2 : Constant  Value=0
  Dot Product : DotProduct  OutDataTypeStr=Inherit: Inherit via internal rule
  Dot Product1 : DotProduct  OutDataTypeStr=Inherit: Inherit via internal rule
  Simulink-PS Converter2 : nesl_utility/Simulink-PS Converter  PhysicalDomain=network_engine_domain  SubClassName=ps_input  LeftPortType=input  RightPortType=output  PseudoPeriodic=off  Frequencies=[]  NoiseDistribution=none  NoiseParameters=[]  Unit=1  AffineConversion=off  FilteringAndDerivatives=filter  SimscapeFilterOrder=1  InputFilterTimeConstant=0.001  UdotUserProvided=0
  Solar Panel1 : Subsystem  mask(Solar Panel){}
      mask help: Models a solar panel using a parallel-connected string of solar cells. The solar cell strings are modeled using a single Solar Cell block from the Simscape(TM) Electrical(TM) Sources library.
      mask Display: image('ee_solar_panel_icon.jpg')
  Switch : Switch  Criteria=u2 > Threshold  SaturateOnIntegerOverflow=off  InputSameDT=off
  + : PMIOPort  Side=Right
  - : PMIOPort  Port=2  Side=Right
  wires:
  Bus Selector1/1 -> Dot Product1/2  "<sun2bodyVec>"
  irradiance/1 -> Bus Selector1/1  "irradience"
  Dot Product/1 -> Switch/1
  Constant2/1 -> Switch/3
  Switch/1 -> Simulink-PS Converter2/1
  Dot Product1/1 -> Dot Product/1
  Constant/1 -> Dot Product1/1
  Bus Selector1/3 -> Switch/2  "<eclipse>"
  Bus Selector1/2 -> Dot Product/2  "<Irradience>"
  connections:
  Solar Panel1/RConn2 -- -/RConn1
  +/RConn1 -- Solar Panel1/RConn1
  Solar Panel1/LConn1 -- Simulink-PS Converter2/RConn1

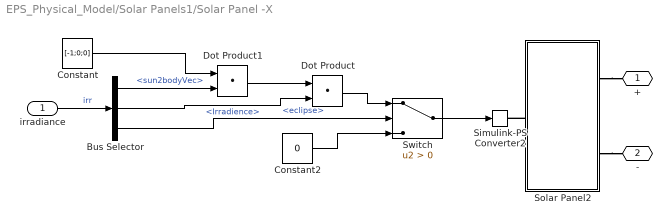
== system EPS_Physical_Model/Solar Panels1/Solar Panel -X ==
  irradiance : Inport
  Bus Selector : BusSelector  OutputSignals=sun2bodyVec,Irradience,eclipse
  Constant : Constant  Value=[-1;0;0]
  Constant2 : Constant  Value=0
  Dot Product : DotProduct  OutDataTypeStr=Inherit: Inherit via internal rule
  Dot Product1 : DotProduct  OutDataTypeStr=Inherit: Inherit via internal rule
  Simulink-PS Converter2 : nesl_utility/Simulink-PS Converter  PhysicalDomain=network_engine_domain  SubClassName=ps_input  LeftPortType=input  RightPortType=output  PseudoPeriodic=off  Frequencies=[]  NoiseDistribution=none  NoiseParameters=[]  Unit=1  AffineConversion=off  FilteringAndDerivatives=filter  SimscapeFilterOrder=1  InputFilterTimeConstant=0.001  UdotUserProvided=0
  Solar Panel2 : Subsystem  mask(Solar Panel){}
      mask help: Models a solar panel using a parallel-connected string of solar cells. The solar cell strings are modeled using a single Solar Cell block from the Simscape(TM) Electrical(TM) Sources library.
      mask Display: image('ee_solar_panel_icon.jpg')
  Switch : Switch  Criteria=u2 > Threshold  SaturateOnIntegerOverflow=off  InputSameDT=off
  + : PMIOPort  Side=Right
  - : PMIOPort  Port=2  Side=Right
  wires:
  irradiance/1 -> Bus Selector/1  "irr"
  Bus Selector/1 -> Dot Product1/2  "<sun2bodyVec>"
  Dot Product/1 -> Switch/1
  Constant2/1 -> Switch/3
  Switch/1 -> Simulink-PS Converter2/1
  Dot Product1/1 -> Dot Product/1
  Constant/1 -> Dot Product1/1
  Bus Selector/3 -> Switch/2  "<eclipse>"
  Bus Selector/2 -> Dot Product/2  "<Irradience>"
  connections:
  Solar Panel2/RConn1 -- +/RConn1
  Solar Panel2/RConn2 -- -/RConn1
  Solar Panel2/LConn1 -- Simulink-PS Converter2/RConn1

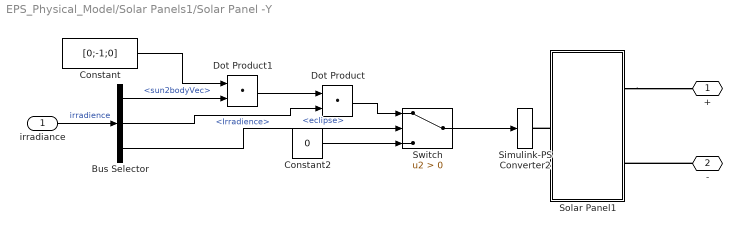
== system EPS_Physical_Model/Solar Panels1/Solar Panel -Y ==
  irradiance : Inport
  Bus Selector : BusSelector  OutputSignals=sun2bodyVec,Irradience,eclipse
  Constant : Constant  Value=[0;-1;0]
  Constant2 : Constant  Value=0
  Dot Product : DotProduct  OutDataTypeStr=Inherit: Inherit via internal rule
  Dot Product1 : DotProduct  OutDataTypeStr=Inherit: Inherit via internal rule
  Simulink-PS Converter2 : nesl_utility/Simulink-PS Converter  PhysicalDomain=network_engine_domain  SubClassName=ps_input  LeftPortType=input  RightPortType=output  PseudoPeriodic=off  Frequencies=[]  NoiseDistribution=none  NoiseParameters=[]  Unit=1  AffineConversion=off  FilteringAndDerivatives=filter  SimscapeFilterOrder=1  InputFilterTimeConstant=0.001  UdotUserProvided=0
  Solar Panel1 : Subsystem  mask(Solar Panel){}
      mask help: Models a solar panel using a parallel-connected string of solar cells. The solar cell strings are modeled using a single Solar Cell block from the Simscape(TM) Electrical(TM) Sources library.
      mask Display: image('ee_solar_panel_icon.jpg')
  Switch : Switch  Criteria=u2 > Threshold  SaturateOnIntegerOverflow=off  InputSameDT=off
  + : PMIOPort  Side=Right
  - : PMIOPort  Port=2  Side=Right
  wires:
  Bus Selector/1 -> Dot Product1/2  "<sun2bodyVec>"
  irradiance/1 -> Bus Selector/1  "irradience"
  Dot Product/1 -> Switch/1
  Constant2/1 -> Switch/3
  Switch/1 -> Simulink-PS Converter2/1
  Dot Product1/1 -> Dot Product/1
  Constant/1 -> Dot Product1/1
  Bus Selector/3 -> Switch/2  "<eclipse>"
  Bus Selector/2 -> Dot Product/2  "<Irradience>"
  connections:
  -/RConn1 -- Solar Panel1/RConn2
  Solar Panel1/RConn1 -- +/RConn1
  Solar Panel1/LConn1 -- Simulink-PS Converter2/RConn1

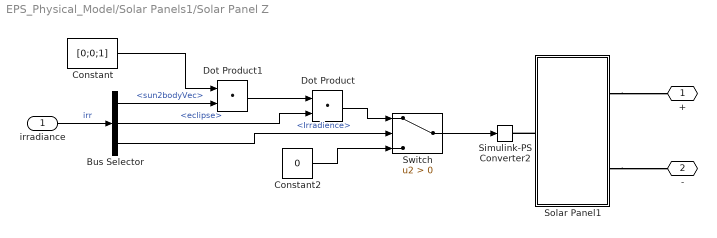
== system EPS_Physical_Model/Solar Panels1/Solar Panel Z ==
  irradiance : Inport
  Bus Selector : BusSelector  OutputSignals=sun2bodyVec,eclipse,Irradience
  Constant : Constant  Value=[0;0;1]
  Constant2 : Constant  Value=0
  Dot Product : DotProduct  OutDataTypeStr=Inherit: Inherit via internal rule
  Dot Product1 : DotProduct  OutDataTypeStr=Inherit: Inherit via internal rule
  Simulink-PS Converter2 : nesl_utility/Simulink-PS Converter  PhysicalDomain=network_engine_domain  SubClassName=ps_input  LeftPortType=input  RightPortType=output  PseudoPeriodic=off  Frequencies=[]  NoiseDistribution=none  NoiseParameters=[]  Unit=1  AffineConversion=off  FilteringAndDerivatives=filter  SimscapeFilterOrder=1  InputFilterTimeConstant=0.001  UdotUserProvided=0
  Solar Panel1 : Subsystem  mask(Solar Panel){}
      mask help: Models a solar panel using a parallel-connected string of solar cells. The solar cell strings are modeled using a single Solar Cell block from the Simscape(TM) Electrical(TM) Sources library.
      mask Display: image('ee_solar_panel_icon.jpg')
  Switch : Switch  Criteria=u2 > Threshold  SaturateOnIntegerOverflow=off  InputSameDT=off
  + : PMIOPort  Side=Right
  - : PMIOPort  Port=2  Side=Right
  wires:
  Bus Selector/2 -> Dot Product/2  "<eclipse>"
  Bus Selector/1 -> Dot Product1/2  "<sun2bodyVec>"
  irradiance/1 -> Bus Selector/1  "irr"
  Dot Product/1 -> Switch/1
  Constant2/1 -> Switch/3
  Switch/1 -> Simulink-PS Converter2/1
  Dot Product1/1 -> Dot Product/1
  Constant/1 -> Dot Product1/1
  Bus Selector/3 -> Switch/2  "<Irradience>"
  connections:
  Solar Panel1/RConn2 -- -/RConn1
  Solar Panel1/RConn1 -- +/RConn1
  Solar Panel1/LConn1 -- Simulink-PS Converter2/RConn1

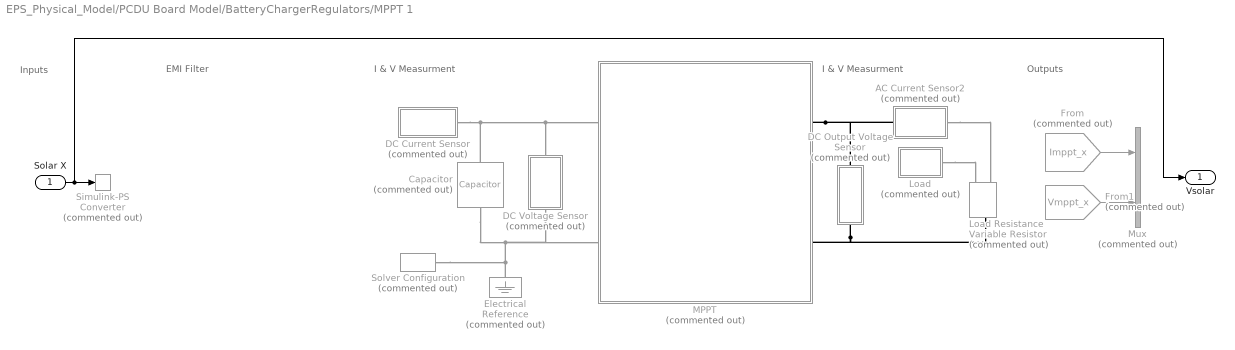
== system EPS_Physical_Model/PCDU Board Model/BatteryChargerRegulators/MPPT 1 ==
  note: I & V Measurment
  note: EMI Filter
  note: I & V Measurment
  note: Inputs
  note: Outputs
  Solar X : Inport
  AC Current Sensor2 : Subsystem  Commented=on
      mask Display: disp('i');
  Capacitor : fl_lib/Electrical/Electrical Elements/Capacitor  Commented=on  c=boost.inputCapacitor F  r=1e-6 Ohm  g=0 1/Ohm  i_specify=off  i_priority=None  i=0 A  i_nominal_specify=off  i_nominal_value=1  i_nominal_unit=A  v_specify=off  v_priority=None  v=solarPlant.startMPPTValue V  v_nominal_specify=off  v_nominal_value=1  v_nominal_unit=V  vc_specify=on  vc_priority=High  vc=solarPlant.startMPPTValue V  vc_nominal_specify=off  vc_nominal_value=1  vc_nominal_unit=V
  DC Current Sensor : Subsystem  Commented=on
      mask Display: disp('i')
  DC Output Voltage Sensor : Subsystem  Commented=on
      mask Display: disp('v')
  DC Voltage Sensor : Subsystem  Commented=on
      mask Display: disp('v');
  Electrical Reference : fl_lib/Electrical/Electrical Elements/Electrical Reference  Commented=on
  From : From  Commented=on  GotoTag=Imppt_x  TagVisibility=global
  From1 : From  Commented=on  GotoTag=Vmppt_x  TagVisibility=global
  Load : Subsystem  Commented=on
  Load Resistance : fl_lib/Electrical/Electrical Elements/Variable Resistor  Commented=on  Rmin=0 Ohm  thermalEnable=false  thermal_mass=1 J/K  i_specify=off  i_priority=None  i=5 A  i_nominal_specify=off  i_nominal_value=1  i_nominal_unit=A  v_specify=off  v_priority=None  v=0 V  v_nominal_specify=off  v_nominal_value=1  v_nominal_unit=V  T_specify=off  T_priority=None  T=300 K  T_nominal_specify=off  T_nominal_value=1  T_nominal_unit=K
  MPPT : Subsystem  Commented=on
  Mux : Mux  Commented=on  Inputs=2
  Simulink-PS Converter : nesl_utility/Simulink-PS Converter  Commented=on  PhysicalDomain=network_engine_domain  SubClassName=ps_input  LeftPortType=input  RightPortType=output  PseudoPeriodic=off  Frequencies=[]  NoiseDistribution=none  NoiseParameters=[]  Unit=1  AffineConversion=off  FilteringAndDerivatives=provide  SimscapeFilterOrder=1  InputFilterTimeConstant=0.001  UdotUserProvided=0
  Solver Configuration : nesl_utility/Solver Configuration  Commented=on  PhysicalDomain=network_engine_domain  SubClassName=solver  LeftPortType=input  RightPortType=generic  Tones=[]  Harmonics=[]  SimulateNoise=off  Profile=off  UseLocalSampling=off  EnableSwitchedLinearOptims=on  FrequencyDomain=off  UseCCode=off  RelTol=0.001  AbsTol=1e-06  MinStep=1e-09  ToWorkspace=off  RevertToSquareIcSolve=off  NumHomotopyIterations=100  PhasorMode=off  PhasorModeNumHarmonics=1  ConsistencySolver=NEWTON_FTOL  IndexReductionMethod=DerivativeReplacement  DoDC=off  ResidualTolerance=1e-9  ConsistencyTolSource=GLOBAL  ConsistencyAbsTol=0.001  ConsistencyRelTol=0.001  ConsistencyTolFactor=0.001  UseLocalSolver=off  LocalSolverChoice=NE_BACKWARD_EULER_ADVANCER  ResolveIndetEquations=on  FunctionEvalNumThread=1  LocalSolverSampleTime=1e-6  DoFixedCost=off  MaxNonlinIter=10  MaxModeIter=2  ComputeImpulses=off  ImpulseIterations=2  LinearAlgebra=auto  LinearAlgebraNumThread=0  EquationFormulation=NE_TIME_EF  DelaysMemoryBudget=1024  AutomaticFiltering=on  FilteringTimeConstant=0.001  PartitionStorageMethod=AS_NEEDED  PartitionMemoryBudget=1024  PartitionMethod=FAST  MultibodyUseLocalSolver=off  MultibodyLocalSolverChoice=ODE1  MultibodyLocalSolverSampleTime=0.001
  Vsolar : Outport
  wires:
  From1/1 -> Mux/2
  From/1 -> Mux/1
  Solar X/1 -> Simulink-PS Converter/1, Vsolar/1
  connections:
  Load/RConn1 -- Load Resistance/LConn1
  AC Current Sensor2/LConn1 -- Load Resistance/LConn2
  MPPT/RConn1 -- AC Current Sensor2/RConn1 -- DC Output Voltage Sensor/RConn1
  DC Output Voltage Sensor/LConn1 -- MPPT/RConn2 -- Load Resistance/RConn1
  Capacitor/LConn1 -- MPPT/LConn1 -- DC Voltage Sensor/RConn1 -- DC Current Sensor/LConn1
  Electrical Reference/LConn1 -- MPPT/LConn2 -- DC Voltage Sensor/LConn1 -- Capacitor/RConn1 -- Solver Configuration/RConn1

== system EPS_Physical_Model/PCDU Board Model/BatteryChargerRegulators/MPPT 2 ==
  Solar Y : Inport
  EMI Filters : Subsystem
  I & V Measurment : Subsystem
  I & V Measurment1 : Subsystem
  MPPT : Subsystem
  Vsolar : Outport
  wires:
  EMI Filters/1(Solar X) -> I & V Measurment/1(Solar X)
  I & V Measurment/1(V solar) -> MPPT/1(In1)
  MPPT/1(Out1) -> I & V Measurment1/1(In1)
  Solar Y/1 -> EMI Filters/1(In1)
  I & V Measurment1/1(V solar) -> Vsolar/1

== system EPS_Physical_Model/PCDU Board Model/BatteryChargerRegulators/MPPT 3 ==
  Solar Z : Inport
  EMI Filters : Subsystem
  I & V Measurment : Subsystem
  I & V Measurment1 : Subsystem
  MPPT : Subsystem
  Vsolar : Outport
  wires:
  EMI Filters/1(Solar X) -> I & V Measurment/1(Solar X)
  I & V Measurment/1(V solar) -> MPPT/1(In1)
  MPPT/1(Out1) -> I & V Measurment1/1(In1)
  Solar Z/1 -> EMI Filters/1(In1)
  I & V Measurment1/1(V solar) -> Vsolar/1

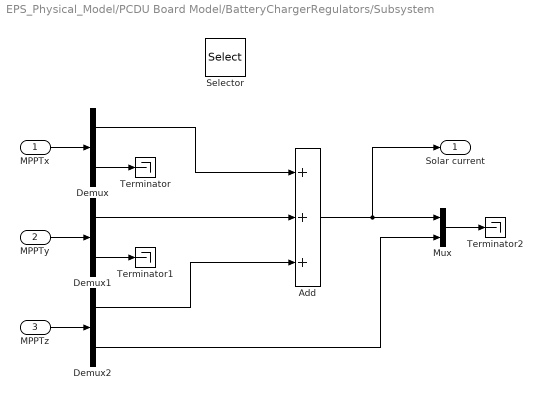
== system EPS_Physical_Model/PCDU Board Model/BatteryChargerRegulators/Subsystem ==
  MPPTx : Inport
  MPPTy : Inport  Port=2
  MPPTz : Inport  Port=3
  Add : Sum  Inputs=+++
  Demux : Demux  Outputs=2
  Demux1 : Demux  Outputs=2
  Demux2 : Demux  Outputs=2
  Mux : Mux  Inputs=2
  Selector : Selector  InputPortWidth=3  IndexOptions=Index vector (dialog)  Indices=[1 3]  OutputSizes=1
  Terminator : Terminator
  Terminator1 : Terminator
  Terminator2 : Terminator
  Solar current : Outport
  wires:
  Mux/1 -> Terminator2/1
  Demux1/2 -> Terminator1/1
  Demux/2 -> Terminator/1
  Demux/1 -> Add/1
  Demux2/2 -> Mux/2
  Add/1 -> Mux/1, Solar current/1
  Demux2/1 -> Add/3
  Demux1/1 -> Add/2
  MPPTz/1 -> Demux2/1
  MPPTy/1 -> Demux1/1
  MPPTx/1 -> Demux/1

== system EPS_Physical_Model/PCDU Board Model/PowerConversionModules/Boost_12V ==
  BatteryVoltage : Inport
  Gain : Gain  Gain=12/6.5
  12V : Outport
  wires:
  Gain/1 -> 12V/1
  BatteryVoltage/1 -> Gain/1

== system EPS_Physical_Model/PCDU Board Model/PowerConversionModules/Boost_3.3V ==
  BatteryVoltage : Inport
  Gain : Gain  Gain=3.3/6.5
  12V : Outport
  wires:
  Gain/1 -> 12V/1
  BatteryVoltage/1 -> Gain/1

== system EPS_Physical_Model/PCDU Board Model/PowerConversionModules/Boost_5V ==
  BatteryVoltage : Inport
  Gain : Gain  Gain=5/6.5
  12V : Outport
  wires:
  BatteryVoltage/1 -> Gain/1
  Gain/1 -> 12V/1

== system EPS_Physical_Model/Solar Panels1/Solar Panel +X/Solar Panel1 ==
  Current-Controlled Current Source : fl_lib/Electrical/Electrical Sources/Current-Controlled Current Source  K=-1  i1_specify=off  i1_priority=None  i1=0 A  i1_nominal_specify=off  i1_nominal_value=1  i1_nominal_unit=A  i2_specify=off  i2_priority=None  i2=0 A  i2_nominal_specify=off  i2_nominal_value=1  i2_nominal_unit=A
      settings: InternalSimscapePortConfiguration="{\"Bottom\":[],\"Left\":[{\"id\":\"p1\",\"label\":\"+\",\"type\":\"foundation.electrical.electrical\"},{\"id\":\"head\",\"label\":\"\",\"type\":\"foundation.electrical.electrical\"}],\"Right\":[{\"id\":\"n1\",\"label\":\"-\",\"type\":\"foundation.electrical.electrical\"},{\"id\":\"tail\",\"label\":\"\",\"type\":\"foundation.electrical.electrical\"}],\"Top\":[]}"
  Solar Cell : ee_lib/Sources/Solar Cell  PartSpecification="{\"DatasetId\":\"AzurSpace|3C44_30sqmm|simscape.electrical.solarCell\",\"DisplayName\":\"AzurSpace:3C44_30sqmm\"}"  prm=3  Isc=1.19 % Datasheet derived A  Voc=3.08 % Datasheet derived V  Is=2.73592960844769e-35 % Datasheet derived A  Is2=1.16779785679844e-37 % Datasheet derived A  Iph=1.19000472592367 % Datasheet derived A  Ir0=250000 % Datasheet derived W/m^2  ec=1.50303550965723 % Datasheet derived  N2=1.59525933684062 % Datasheet derived  Rs=0.104281524604326 % Datasheet derived Ohm  Rp=26248.1045129446 % Datasheet derived Ohm  N_series=1 % Datasheet derived  N_parallel=1 % Datasheet derived  TIPH1=0.000799987520460482 % Datasheet derived 1/K  EG=1.441 % Datasheet derived eV  TXIS1=92.8777524632801 % Datasheet derived  TXIS2=227.92622072394 % Datasheet derived  TRS1=0.0216421647602992 % Datasheet derived  TRP1=0 % Parameter not set  Tmeas=25 % Datasheet derived degC  TFIXED=25 % Datasheet derived degC  thermal_mass=100 % Parameter not set J/K  initial_temperature=25 degC
      settings: AttributesFormatString=AzurSpace:3C44_30sqmm
  Ir : PMIOPort  Side=Left
  + : PMIOPort  Port=2  Side=Right
  - : PMIOPort  Port=3  Side=Right
  connections:
  Current-Controlled Current Source/LConn2 -- -/RConn1 -- Solar Cell/RConn1
  Ir/RConn1 -- Solar Cell/LConn1
  Current-Controlled Current Source/LConn1 -- Solar Cell/LConn2
  Current-Controlled Current Source/RConn1 -- Current-Controlled Current Source/RConn2 -- +/RConn1
